simulink model "lab_2a"  (R2020a)
settings: Solver=VariableStepAuto  StartTime=0.0  StopTime=10  RelTol=1e-3
libraries: powerlib x32
settings Model: Creator=Dhanush Wagle  LastModifiedBy=Dhanush Wagle

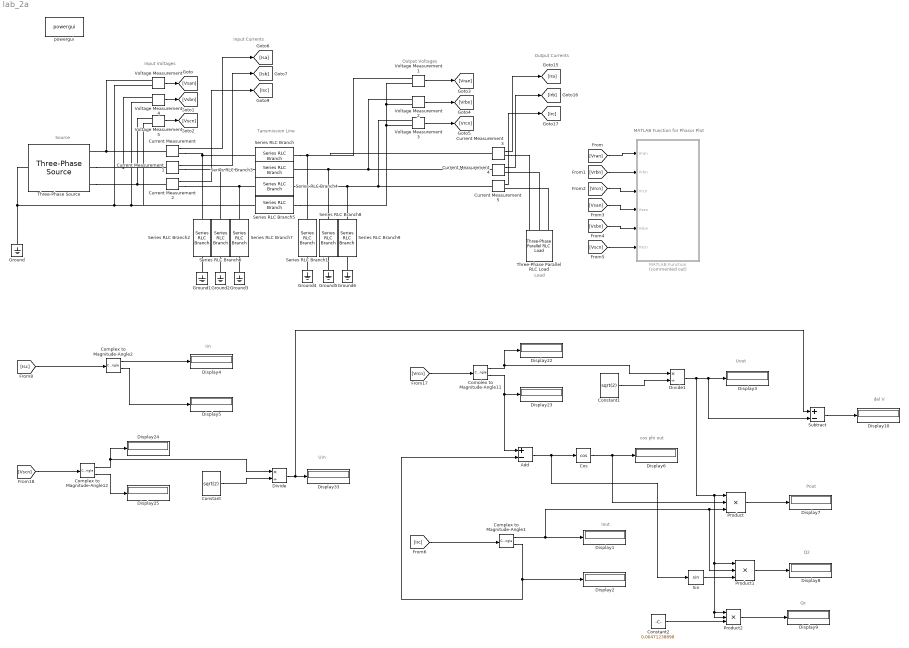
== system lab_2a ==
  note: del V
  note: Qc
  note: Q2
  note: Pout
  note: cos phi out
  note: Iout
  note: Uout
  note: Uin
  note: Iin
  note: MATLAB Function for Phasor Plot
  note: Output Currents
  note: Output Voltages
  note: Input Currents
  note: Input Voltages
  note: Tansmission Line
  note: Load
  note: Source
  Add : Sum  Inputs=+-
  Complex to Magnitude-Angle{1..2,11..12} (4 alike) : ComplexToMagnitudeAngle
  Constant : Constant  Value=sqrt(2)
  Constant1 : Constant  Value=sqrt(2)
  Constant2 : Constant  Value=0.00471238898
  Cos : Trigonometry  Operator=cos
  Current Measurement{,1..5} (6 alike) : powerlib/Measurements/Current Measurement  PhasorSimulation=on  OutputType=Complex  PSBequivalent=0
  Display{1..10,22..25,33} (15 alike) : Display
  Divide : Product  Inputs=*/
  Divide1 : Product  Inputs=*/
  Ground{,1..6} (7 alike) : powerlib/Elements/Ground  LConnTagsString=a
  MATLAB Function : MATLAB Function  Commented=on  TreatAsAtomicUnit=on
  Product : Product  Inputs=3
  Product1 : Product  Inputs=3
  Product2 : Product  Inputs=3
  Series RLC Branch{,3..5} (4 alike) : powerlib/Elements/Series RLC Branch  LConnTagsString=__new0  RConnTagsString=__new0  BranchType=RL  Resistance=2.12  Inductance=0.0112687  SetiL0=off  InitialCurrent=0  Capacitance=13.6e-6  Setx0=off  InitialVoltage=0  Measurements=None
  Series RLC Branch{1..2,6..9} (6 alike) : powerlib/Elements/Series RLC Branch  LConnTagsString=__new0  RConnTagsString=__new0  BranchType=C  Resistance=1  Inductance=1e-3  SetiL0=off  InitialCurrent=0  Capacitance=15e-6  Setx0=off  InitialVoltage=0  Measurements=None
  Sin : Trigonometry
  Subtract : Sum  Inputs=+-
  Three-Phase Parallel RLC Load : powerlib/Elements/Three-Phase Parallel RLC Load  LConnTagsString=A|B|C  Configuration=Y (grounded)  NominalVoltage=117.4  Vabc=[120 120 120]  Vabcp=[1e3 1e3 1e3]  NominalFrequency=50  UnbalancedPower=on  ActivePower=265.324  InductivePower=0  CapacitivePower=0  Pabc=[265 265 265]  QLabc=[0 0 0]  QCabc=[0 0 0]  Pabcp=[10e3 9e3 11e3]  QLabcp=0  QCabcp=0  Measurements=None  LoadType=constant Z
  Three-Phase Source : powerlib/Electrical Sources/Three-Phase Source  InternalConnection=Yn  VoltagePhases=on  Voltage=120  PhaseAngle=0  Voltage_phases=[120 120 120]  PhaseAngles_phases=[0 -120 +120]  Frequency=50  NonIdealSource=on  SpecifyImpedance=off  Resistance=0.000001  Inductance=16.58e-9  ShortCircuitLevel=100e6  BaseVoltage=230  XRratio=7  BusType=swing  Pref=10e3  Qref=0  Prefabc=[10e3, 10e3, 10e3]  Qrefabc=[0, 0, 0]  Qmin=-inf  Qmax=inf
  Voltage Measurement{,1..5} (6 alike) : powerlib/Measurements/Voltage Measurement  PhasorSimulation=on  OutputType=Complex  PSBequivalent=0
  powergui : powerlib/powergui  Priority=1  SimulationMode=Phasor  SampleTime=50e-6  frequency=50  Iterations=50  frequencyindice=50  Pbase=100e6  ErrMax=1e-4  UnitsV=kV  UnitsW=MW  buscounter=0  FunctionMessages=off  echomessages=off  EnableUseOfTLC=off  CurrentSourceSwitches=off  DisableSnubberDevices=off  DisableRonSwitches=off  DisableVfSwitches=off  DisplayEquations=off  AutomaticDiscreteSolvers=off  SolverType=Tustin/Backward Euler (TBE)  Interpol=off  ExternalGateDelay=off  methode=off  Ts=100  x0status=blocks  SPID=on  SwTol=0  HookPort=off  NonlinearTolerance=1e-4  nMaxIteration=100  ContinueOnMaxIteration=off  RestoreLinks=warning  ResistiveCurrentMeasurement=off  Frange=[0:2:500]  Ylog=off  Xlog=on  ShowGrid=off  save=off  variable=ZData  structure=0  ZoomFFT=off  StartTime=0.0  cycles=1  DisplayStyle=1  fundamental=60  FreqAxis=off  MaxFrequency=1000  frequencyindicesteady=1  RmsSteady=1  display=off
  wires:
  Voltage Measurement/1 -> [Vsan]
  Voltage Measurement4/1 -> [Vsbn]
  Voltage Measurement5/1 -> [Vscn]
  Voltage Measurement1/1 -> [Vran]
  Voltage Measurement2/1 -> [Vrbn]
  Voltage Measurement3/1 -> [Vrcn]
  [Vran] -> MATLAB Function/1(Vran)
  [Vrbn] -> MATLAB Function/2(Vrbn)
  [Vrcn] -> MATLAB Function/3(Vrcn)
  [Vsan] -> MATLAB Function/4(Vsan)
  [Vsbn] -> MATLAB Function/5(Vsbn)
  [Vscn] -> MATLAB Function/6(Vscn)
  Current Measurement/1 -> [Isa]
  Current Measurement1/1 -> [Isb]
  Current Measurement2/1 -> [Isc]
  [Isc] -> Complex to Magnitude-Angle2/1
  Complex to Magnitude-Angle2/2 -> Display5/1
  Complex to Magnitude-Angle2/1 -> Display4/1
  [Vrcn] -> Complex to Magnitude-Angle11/1
  Complex to Magnitude-Angle11/2 -> Add/1, Display23/1
  [Vscn] -> Complex to Magnitude-Angle12/1
  Complex to Magnitude-Angle12/1 -> Divide/1, Display24/1
  Complex to Magnitude-Angle12/2 -> Display25/1
  Current Measurement3/1 -> [Ira]
  Current Measurement4/1 -> [Irb]
  Current Measurement5/1 -> [Irc]
  Divide/1 -> Subtract/1, Display33/1
  Constant/1 -> Divide/2
  Complex to Magnitude-Angle1/1 -> Product1/2, Product/3, Display1/1
  [Irc] -> Complex to Magnitude-Angle1/1
  Complex to Magnitude-Angle1/2 -> Display2/1, Add/2
  Complex to Magnitude-Angle11/1 -> Display22/1, Divide1/1
  Divide1/1 -> Product2/2, Product2/1, Product1/1, Product/1, Subtract/2, Display3/1
  Constant1/1 -> Divide1/2
  Add/1 -> Sin/1, Cos/1
  Cos/1 -> Product/2, Display6/1
  Product/1 -> Display7/1
  Sin/1 -> Product1/3
  Product1/1 -> Display8/1
  Product2/1 -> Display9/1
  Constant2/1 -> Product2/3
  Subtract/1 -> Display10/1
  connections:
  Current Measurement/RConn1 -- Series RLC Branch2/LConn1 -- Series RLC Branch/LConn1
  Series RLC Branch/RConn1 -- Voltage Measurement1/LConn1 -- Current Measurement3/LConn1 -- Series RLC Branch1/LConn1
  Series RLC Branch5/LConn1 -- Voltage Measurement5/LConn2 -- Voltage Measurement4/LConn2 -- Voltage Measurement/LConn2 -- Three-Phase Source/LConn1 -- Ground/LConn1
  Series RLC Branch6/LConn1 -- Current Measurement1/RConn1 -- Series RLC Branch3/LConn1
  Series RLC Branch7/LConn1 -- Current Measurement2/RConn1 -- Series RLC Branch4/LConn1
  Voltage Measurement3/LConn1 -- Current Measurement5/LConn1 -- Series RLC Branch4/RConn1 -- Series RLC Branch9/LConn1
  Ground1/LConn1 -- Series RLC Branch2/RConn1
  Ground2/LConn1 -- Series RLC Branch6/RConn1
  Ground3/LConn1 -- Series RLC Branch7/RConn1
  Ground4/LConn1 -- Series RLC Branch1/RConn1
  Ground5/LConn1 -- Series RLC Branch8/RConn1
  Ground6/LConn1 -- Series RLC Branch9/RConn1
  Voltage Measurement3/LConn2 -- Series RLC Branch5/RConn1 -- Voltage Measurement2/LConn2 -- Voltage Measurement1/LConn2
  Three-Phase Source/RConn2 -- Current Measurement1/LConn1 -- Voltage Measurement4/LConn1
  Voltage Measurement/LConn1 -- Current Measurement/LConn1 -- Three-Phase Source/RConn1
  Three-Phase Source/RConn3 -- Voltage Measurement5/LConn1 -- Current Measurement2/LConn1
  Voltage Measurement2/LConn1 -- Current Measurement4/LConn1 -- Series RLC Branch8/LConn1 -- Series RLC Branch3/RConn1
  Three-Phase Parallel RLC Load/LConn2 -- Current Measurement4/RConn1
  Three-Phase Parallel RLC Load/LConn3 -- Current Measurement5/RConn1
  Current Measurement3/RConn1 -- Three-Phase Parallel RLC Load/LConn1

== matlab function lab_2a/MATLAB Function ==
  data: Vran input; Vrbn input; Vrcn input; Vsan input; Vsbn input; Vscn input
function plot(Vran, Vrbn, Vrcn, Vsan, Vsbn, Vscn)

Vran = Vran/sqrt(3);
Vrbn = Vrbn/sqrt(3);
Vrcn = Vrcn/sqrt(3);
Vsan = Vsan/sqrt(3);
Vsbn = Vsbn/sqrt(3);
Vscn = Vscn/sqrt(3);

angle1 = angle(Vran)*ones(1,10);
angle2 = angle(Vrbn)*ones(1,10);
angle3 = angle(Vrcn)*ones(1,10);
angle4 = angle(Vsan)*ones(1,10);
angle5 = angle(Vsbn)*ones(1,10);
angle6 = angle(Vscn)*ones(1,10);

value1 = linspace(0, abs(Vran), 10);
value2 = linspace(0, abs(Vrbn), 10);
value3 = linspace(0, abs(Vrcn), 10);
value4 = linspace(0, abs(Vsan), 10);
value5 = linspace(0, abs(Vsbn), 10);
value6 = linspace(0, abs(Vscn), 10);

figure(1)
polar(angle1, value1, 'r');

hold on

polar(angle2, value2, 'y');
polar(angle3, value3, 'b');
polar(angle4, value4, 'r');
polar(angle5, value5, 'y');
polar(angle6, value6, 'b');

function set_text(V, T, ang)
text(cos(angle(V)+ang)*abs(V), sin(angle(V)+ang)*abs(V), T)
end

set_text(Vran, 'Vran', 0.05)
set_text(Vrbn, 'Vrbn', 0.05)
set_text(Vrcn, 'Vrcn', 0.05)
set_text(Vsan, 'Vsan', 0.05)
set_text(Vsbn, 'Vsbn', 0.05)
set_text(Vscn, 'Vscn', 0.05)

end
